simulink model "SIRek"  (Simulink 7.9)
settings: Solver=ode45  StartTime=0.0  StopTime=t  RelTol=1e-3
values from neighbouring files (symbols this model uses):
  beta = 0.7    [SEIR.m]    (also in SI.m = 0.1; SIR.m = 0.4; modele_epidemiologiczne.m = str2num(get(handles.edit6, 'String')))
  I0 = str2num(get(handles.edit3, 'String'))    [modele_epidemiologiczne.m]
  lambda = 0.01    [SEIR.m]    (also in SIR.m = 0.1; modele_epidemiologiczne.m = str2num(get(handles.edit8, 'String')))
  R0 = str2num(get(handles.edit1, 'String'))    [modele_epidemiologiczne.m]
  S0 = str2num(get(handles.edit4, 'String'))    [modele_epidemiologiczne.m]
settings Model: Creator=grzesiek  LastModifiedBy=Zaneta
settings DebuggingCC: FcnCallInpInsideContextMsg=Use local settings  StrictBusMsg=Warning
settings GRTTargetCC: CombineOutputUpdateFcns=off  GRTInterface=on

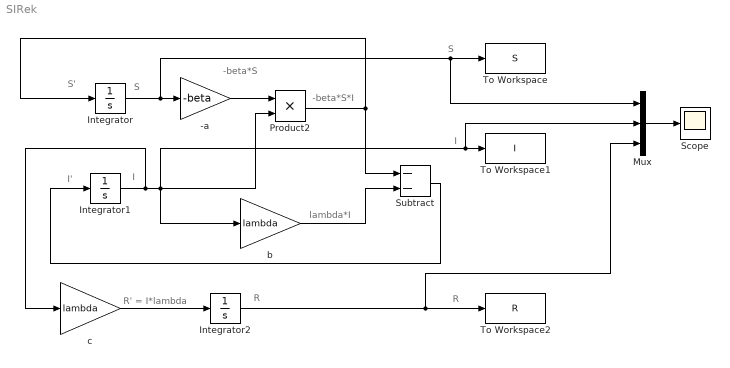
== system SIRek ==
  note: S
  note: R
  note: I
  note: I'
  note: S'
  note: R' = I*lambda
  note: -beta*S*I
  note: S
  note: I
  note: R
  note: -beta*S
  note: lambda*I
  -a : Gain  Gain=-beta
  Integrator : Integrator  InitialCondition=S0
  Integrator1 : Integrator  InitialCondition=I0
  Integrator2 : Integrator  InitialCondition=R0
  Mux : Mux  Inputs=3
  Product2 : Product  RndMeth=Zero
  Scope : Scope
  Subtract : Sum  Inputs=--
  To Workspace : ToWorkspace  VariableName=S  SampleTime=-1
  To Workspace1 : ToWorkspace  VariableName=I  SampleTime=-1
  To Workspace2 : ToWorkspace  VariableName=R  SampleTime=-1
  b : Gain  Gain=lambda
  c : Gain  Gain=lambda
  wires:
  Integrator/1 -> -a/1, To Workspace/1, Mux/1
  -a/1 -> Product2/1
  Integrator1/1 -> Product2/2, b/1, To Workspace1/1, Mux/2, c/1
  Product2/1 -> Integrator/1, Subtract/1
  b/1 -> Subtract/2
  Subtract/1 -> Integrator1/1
  c/1 -> Integrator2/1
  Integrator2/1 -> To Workspace2/1, Mux/3
  Mux/1 -> Scope/1
